simulink model "Task_20"  (R2022b)
settings: Solver=VariableStepAuto  StartTime=0.0  StopTime=10.0  RelTol=1e-3
settings Model: Creator=Abanob_Sameh  LastModifiedBy=Abanob_Sameh

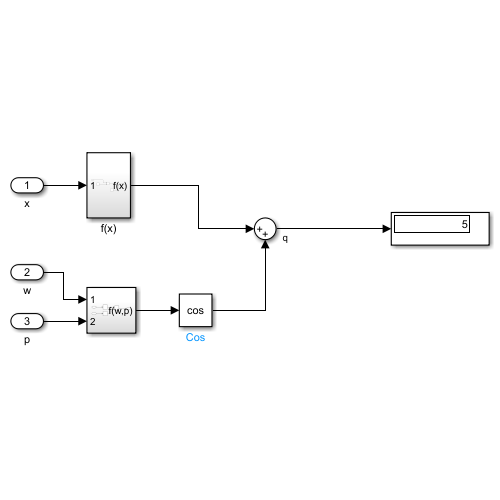
[thumbnail: Simulink's stored preview of the top-level diagram]
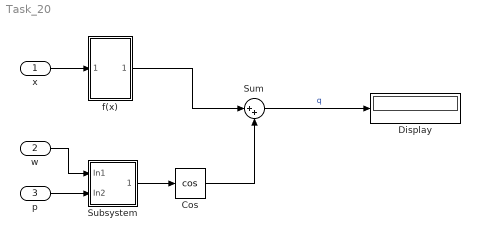
== system Task_20 ==
  x : Inport
  w : Inport  Port=2
  p : Inport  Port=3
  Cos : Trigonometry  Operator=cos
  Display : Display
  Subsystem : Subsystem
  Sum : Sum  Inputs=|++
  f(x) : Subsystem
  wires:
  Subsystem/1(f(w,p)) -> Cos/1
  w/1 -> Subsystem/1(In1)
  p/1 -> Subsystem/2(In2)
  f(x)/1(f(x)) -> Sum/1
  x/1 -> f(x)/1(In1)
  Cos/1 -> Sum/2
  Sum/1 -> Display/1  "q"

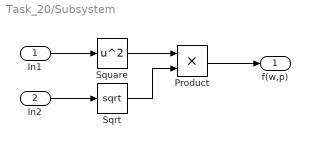
== system Task_20/Subsystem ==
  In1 : Inport
  In2 : Inport  Port=2
  Product : Product
  Sqrt : Sqrt
  Square : Math  Operator=square
  f(w,p) : Outport
  wires:
  Square/1 -> Product/1
  Product/1 -> f(w,p)/1
  In2/1 -> Sqrt/1
  Sqrt/1 -> Product/2
  In1/1 -> Square/1

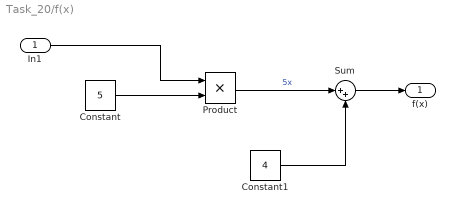
== system Task_20/f(x) ==
  In1 : Inport
  Constant : Constant  Value=5
  Constant1 : Constant  Value=4
  Product : Product
  Sum : Sum  Inputs=|++
  f(x) : Outport
  wires:
  Product/1 -> Sum/1  "5x"
  Constant1/1 -> Sum/2
  In1/1 -> Product/1
  Constant/1 -> Product/2
  Sum/1 -> f(x)/1
